simulink model "UDE_quadrotor"  (R2017b)
settings: Solver=ode4  StartTime=0.0  StopTime=40  FixedStep=0.001  RelTol=1e-3
InitFcn:
  | initial_conditions_and_parameters;
values from neighbouring files (symbols this model uses):
  psi_initial = 0.0    (= 0)    [Parameters_and_initial_conditions.m]
  T_passive = 0.5    [Parameters_and_initial_conditions.m]
  theta_initial = 0.0    (= 0)    [Parameters_and_initial_conditions.m]
undefined symbols (not defined in the file or in its folder): a1_x, a1_y, a1_z, a2_x, a2_y, a2_z, CD, Enable_desired_angular_rate_differentiator, ESC_k, ESC_p, f_g, ftau_b, g, hM, hT, Inner_loop_controller_switch, Ir, kd_h, kd_phi, kd_psi, kd_theta, kd_x, kd_y, kd_z, kp_phi, kp_psi, kp_theta, kp_x, kp_y, kp_z, LT, m, p_initial, phi_initial, q_initial, r_initial, T_dif, T_max, T_phi, T_phi1, T_phi2, T_phi3, T_theta, T_theta1, T_theta2, T_theta3, T_x, T_y, T_z, tau_x_max, tau_y_max, tau_z_max, Tf_x, Tf_y, Tf_z, Tn_h, Tn_x, Tn_y, Tn_z, u_initial ... (+5)
libraries: aerolibanim x1, simulink x1, dspsrcs4 x1
(part 2 of 2)

== system UDE_quadrotor/Y-channel virtual controller (generates desired phi)/UDE_y classic ==
  y_d - y : Inport
  y_d_dot - y_dot : Inport  Port=2
  Gain1 : Gain  Gain=kd_y
  Gain2 : Gain  Gain=-1/T_y
  Gain3 : Gain  Gain=kp_y
  Integrator : Integrator
  Sum6 : Sum  Inputs=+++
  f_hat_y : Outport
  wires:
  y_d - y/1 -> Integrator/1, Gain1/1
  Integrator/1 -> Gain3/1
  Gain1/1 -> Sum6/1
  Sum6/1 -> Gain2/1
  Gain3/1 -> Sum6/2
  Gain2/1 -> f_hat_y/1
  y_d_dot - y_dot/1 -> Sum6/3

== system UDE_quadrotor/Yaw (psi) controller/UDE_psi ==
  note: ftau_yb_hat = - (1/T_theta) * [kd_theta*(theta_d - theta) + kp_theta * integral(theta_d - theta) + (theta_d_dot - theta_dot)]
  theta_d - theta : Inport
  theta_d_dot - theta_dot : Inport  Port=2
  Gain1 : Gain  Gain=kd_theta
  Gain2 : Gain  Gain=-1/T_theta
  Gain3 : Gain  Gain=kp_theta
  Integrator : Integrator
  Sum6 : Sum  Inputs=+++
  ftau_yb_hat : Outport
  wires:
  theta_d_dot - theta_dot/1 -> Sum6/3
  theta_d - theta/1 -> Integrator/1, Gain1/1
  Integrator/1 -> Gain3/1
  Gain1/1 -> Sum6/1
  Sum6/1 -> Gain2/1
  Gain3/1 -> Sum6/2
  Gain2/1 -> ftau_yb_hat/1

== matlab function UDE_quadrotor/Quadrotor Dynamic Model/Coordinate Transformation Ground-frame to Body-frame ==
  data: xg input; yg input; zg input; xb output; yb output; zb output; theta input; phi input; psi input
% ==== coordinate transformation function ====
% 
% ==== variables ====
% theta,phi,psi - Euler angles 
% Vg=[xg;yg;zg] - vector in ground coordinate
% Vb=[xb;yb;zb] - vector in body coordinate
% 
% ==== function ====
% This function transfers Vb to Vg.
% 
% ===== note =====
% 


function [xb,yb,zb] = G_to_B(xg,yg,zg,theta,phi,psi)
  S_trans = zeros(3,3);
  S_trans(1,:) = [cos(psi)*cos(theta), cos(psi)*sin(theta)*sin(phi)-cos(phi)*sin(psi), sin(psi)*sin(phi)+cos(psi)*cos(phi)*sin(theta)];
  S_trans(2,:) = [cos(theta)*sin(psi), cos(psi)*cos(phi)+sin(psi)*sin(theta)*sin(phi), cos(phi)*sin(psi)*sin(theta)-cos(psi)*sin(phi)];
  S_trans(3,:) = [-sin(theta), cos(theta)*sin(phi), cos(theta)*cos(phi)];
  S_trans = S_trans';
  xb = S_trans(1,:)*[xg;yg;zg];
  yb = S_trans(2,:)*[xg;yg;zg];
  zb = S_trans(3,:)*[xg;yg;zg];
end

== matlab function UDE_quadrotor/Quadrotor Dynamic Model/Coordinate Transformation Body-frame to Ground-frame ==
  data: xg output; yg output; zg output; xb input; yb input; zb input; theta input; phi input; psi input
% ==== coordinate transformation function ====
% 
% ==== variables ====
% theta,phi,psi - Euler angles 
% Vg=[xg;yg;zg] - vector in ground coordinate
% Vb=[xb;yb;zb] - vector in body coordinate
% 
% ==== function ====
% This function transfers Vb to Vg.
% 
% ===== note =====
% 


function [xg,yg,zg] = B_to_G(xb,yb,zb,theta,phi,psi)
  S_trans = zeros(3,3);
  S_trans(1,:) = [cos(psi)*cos(theta), cos(psi)*sin(theta)*sin(phi)-cos(phi)*sin(psi), sin(psi)*sin(phi)+cos(psi)*sin(theta)*cos(phi)];
  S_trans(2,:) = [cos(theta)*sin(psi), cos(psi)*cos(phi)+sin(psi)*sin(theta)*sin(phi), sin(psi)*cos(phi)*sin(theta)-cos(psi)*sin(phi)];
  S_trans(3,:) = [-sin(theta), cos(theta)*sin(phi), cos(theta)*cos(phi)];
  xg = S_trans(1,:)*[xb;yb;zb];
  yg = S_trans(2,:)*[xb;yb;zb];
  zg = S_trans(3,:)*[xb;yb;zb];
end

== matlab function UDE_quadrotor/Height controller/convert virtual input u_h to lift command T ==
  data: u_z input; m input; g input; T_cmd output; theta input; phi input
function T_cmd = Conversion_u_z_to_T(u_z,m,g,theta,phi)
T_cmd = (m*g-m*u_z)/(cos(theta)*cos(phi));
end

== matlab function UDE_quadrotor/X-channel virtual controller (generates desired theta)/convert virtual input u_x to desired theta ==
  data: u_x input; m input; T input; phi input; theta_d output; psi input
function theta_d = Conversion_u_x_to_theta_d(u_x,m,T,phi,psi)
k_theta = 1; % k_theta * theta_d = sin(theta)
if (T<5)  % avoid singularity
    T = 5;
end
theta_d =  - m*u_x/(k_theta*T*cos(psi)*cos(phi));
end

== matlab function UDE_quadrotor/Y-channel virtual controller (generates desired phi)/convert virtual input u_y to desired phi ==
  data: u_y input; m input; T input; phi_d output; psi input
function phi_d = Conversion_u_y_to_phi_d(u_y,m,T,psi)
k_phi = 1; % k_phi * phi_d = sin(phi)
if (T<5)  % avoid singularity
    T = 5;
end
phi_d =  m*u_y/(k_phi*T*cos(psi));
end

== matlab function UDE_quadrotor/Quadrotor Dynamic Model/dphi//dt ==
  data: p input; q input; r input; theta input; phi input; dphi output
function dphi = Equation_dphi(p,q,r,theta,phi)
dphi = p + (r*cos(phi)+q*sin(phi))*tan(theta);
end

== matlab function UDE_quadrotor/Quadrotor Dynamic Model/du//dt ==
  data: u input; v input; w input; du output; q input; r input; theta input; CDx input; f_xb input; g input; m input
function du = Equation_du(u,v,w,q,r,theta,CDx,f_xb,g,m)
du = v*r - w*q - g*sin(theta) - CDx*u*abs(u)/m + f_xb/m;
% - CDx*u*abs(u) is the air drag along body-x axis
end

== matlab function UDE_quadrotor/Quadrotor Dynamic Model/dv//dt ==
  data: u input; v input; w input; dv output; p input; r input; theta input; phi input; CDy input; f_yb input; g input; m input
function dv = Equation_dv(u,v,w,p,r,theta,phi,CDy,f_yb,g,m)
dv = -u*r + w*p + g*cos(theta)*sin(phi) - CDy*v*abs(v)/m + f_yb/m;
end

== matlab function UDE_quadrotor/Quadrotor Dynamic Model/dw//dt ==
  data: u input; v input; w input; dw output; p input; q input; theta input; phi input; CDz input; f_zb input; T input; g input; m input
function dw = Equation_dw(u,v,w,p,q,theta,phi,CDz,f_zb,T,g,m)
dw = u*q - v*p + g*cos(theta)*cos(phi) - T/m - CDz*w*abs(w)/m + f_zb/m;
end

== matlab function UDE_quadrotor/Quadrotor Dynamic Model/dp//dt ==
  data: q input; r input; Ix input; Iy input; Iz input; gyroeffect_xb input; dp output; tau_xb input; ftau_xb input
function dp = Equation_dp(q,r,Ix,Iy,Iz,gyroeffect_xb,tau_xb,ftau_xb)
dp = (q*r*(Iy-Iz) + gyroeffect_xb + tau_xb + ftau_xb)/Ix;
end

== matlab function UDE_quadrotor/Quadrotor Dynamic Model/dq//dt ==
  data: p input; r input; Ix input; Iy input; Iz input; gyroeffect_yb input; dq output; tau_yb input; ftau_yb input
function dq = Equation_dq(p,r,Ix,Iy,Iz,gyroeffect_yb,tau_yb,ftau_yb)
dq = (p*r*(Iz-Ix)+ gyroeffect_yb + tau_yb + ftau_yb)/Iy;
end

== matlab function UDE_quadrotor/Quadrotor Dynamic Model/dr//dt ==
  data: p input; q input; Ix input; Iy input; Iz input; gyroeffect_zb input; tau_zb input; dr output; ftau_zb input
function dr = Equation_dr(p,q,Ix,Iy,Iz,gyroeffect_zb,tau_zb,ftau_zb)
dr = (p*q*(Ix-Iy) + gyroeffect_zb + tau_zb + ftau_zb)/Iz;
end

== matlab function UDE_quadrotor/Quadrotor Dynamic Model/dtheta//dt ==
  data: q input; r input; phi input; dtheta output
function dtheta = Equation_dtheta(q,r,phi)
dtheta = q*cos(phi) - r*sin(phi);
end

== matlab function UDE_quadrotor/Quadrotor Dynamic Model/dpsi//dt ==
  data: q input; r input; theta input; phi input; dpsi output
function dpsi = Equation_dpsi(q,r,theta,phi)
dpsi = (r*cos(phi)+q*sin(phi))/cos(theta);
end
